simulink model "mpc_doubleint"  (R2017a)
settings: Solver=ode4  StartTime=0.0  StopTime=23  FixedStep=0.1  RelTol=1e-3
libraries: mpclib x1
settings Model: ExtModeTrigMode=oneshot  ExtModeArmWhenConnect=off  Creator=The MathWorks, Inc.  LastModifiedBy=Administrador
settings DataIOCC: SaveFormat=Array  SaveOutput=off  SignalLogging=off  DSMLogging=off  SaveTime=off  SignalLoggingName=sigsOut
settings OptimizationCC: BooleanDataType=off  DefaultParameterBehavior=Inlined  PassReuseOutputArgsAs=Individual arguments  ExpressionDepthLimit=2147483647  InitFltsAndDblsToZero=on
settings DebuggingCC: SaveWithParameterizedLinksMsg=none  UnderspecifiedInitializationDetection=Classic  MergeDetectMultiDrivingBlocksExec=none  SignalResolutionControl=TryResolveAllWithWarning  MultiTaskDSMMsg=warning  MultiTaskCondExecSysMsg=none  IntegerOverflowMsg=none  ParameterTunabilityLossMsg=error  FcnCallInpInsideContextMsg=warning  StateNameClashWarn=warning  SFUnexpectedBacktrackingDiag=warning  SFNoUnconditionalDefaultTransitionDiag=warning  SFExecutionAtInitializationDiag=none  IntegerSaturationMsg=none
settings HardwareCC: ProdBitPerPointer=32  ProdBitPerSizeT=32  ProdBitPerPtrDiffT=32  ProdLargestAtomicFloat=None  ProdIntDivRoundTo=Undefined  ProdEndianess=Unspecified  ProdWordSize=32  ProdHWDeviceType=32-bit Generic  TargetBitPerPointer=64  TargetBitPerSizeT=64  TargetBitPerPtrDiffT=64  TargetLongLongMode=on  TargetIntDivRoundTo=Zero  TargetEndianess=LittleEndian  TargetWordSize=64  TargetHWDeviceType=MATLAB Host  ProdEqTarget=off
settings ModelReferenceCC: PropagateSignalLabelsOutOfModel=off
settings SFSimCC: MATLABDynamicMemAlloc=off
settings RTWCC: SystemTargetFile=ert.tlc  TemplateMakefile=ert_default_tmf  Description=Embedded Coder  GenerateReport=on  IncludeHyperlinkInReport=on  LaunchReport=on  GenerateTraceInfo=on  GenerateTraceReport=on  GenerateTraceReportSl=on  GenerateTraceReportSf=on  GenerateTraceReportEml=on
settings CodeAppCC: ForceParamTrailComments=on  IgnoreCustomStorageClasses=off  OperatorAnnotations=on  SimulinkDataObjDesc=on  SFDataObjDesc=on  MATLABFcnDesc=on  InsertBlockDesc=on  MATLABSourceComments=on
settings ERTTargetCC: GenerateSampleERTMain=on  SupportContinuousTime=on  InlinedParameterPlacement=NonHierarchical  ERTCustomFileTemplate=example_file_process.tlc
settings ConfigComp: CovMetricSettings=dw  CovHtmlReporting=on  CovSaveCumulativeToWorkspaceVar=on  CovSaveSingleToWorkspaceVar=on  CovExternalEMLEnable=off  CovSFcnEnable=off

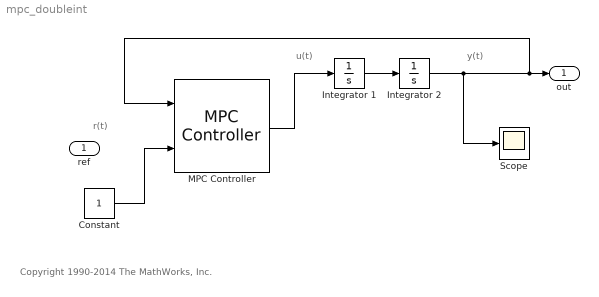
== system mpc_doubleint ==
  note: u(t)
  note: y(t)
  note: r(t)
  note: Copyright 1990-2014 The MathWorks, Inc.
  ref : Inport
  Constant : Constant
  Integrator 1 : Integrator  UpperSaturationLimit=Inf  LowerSaturationLimit=-Inf
  Integrator 2 : Integrator  UpperSaturationLimit=Inf  LowerSaturationLimit=-Inf
  MPC Controller : mpclib/MPC Controller  mpcobj=mpcobj  x0=[]  is_multiple=0  enable_value=0  return_u0=off  ref_from_ws=off  ref_signal_name=[]  ref_preview=on  md_from_ws=off  md_signal_name=[]  md_preview=on  from_project=off  project_file=MPCtask.mat  md_inport=off  mv_inport=off  cost_outport=off  return_sequence=off  return_qpstatus=off  return_state=off  state_inport=off  lims_inport=off  ywt_inport=off  is_designfromscratch=0  uwt_inport=off  duwt_inport=off  rhoeps_inport=off  uref_inport=off  n_ts=0.1  n_mv=1  n_md=0  n_ud=0  n_mo=1  n_uo=0  BlockDataType=double  SampleTimeInherited=off  switch_inport=off
  Scope : Scope
  out : Outport
  wires:
  MPC Controller/1 -> Integrator 1/1
  Integrator 2/1 -> Scope/1, out/1, MPC Controller/1
  Integrator 1/1 -> Integrator 2/1
  Constant/1 -> MPC Controller/2
